simulink model "Starssensegment"  (R2021a)
settings: Solver=VariableStepAuto  StartTime=0.0  StopTime=10  RelTol=1e-3
libraries: simulink x1
settings Model: SnapshotBufferSize=50  SnapshotInterval=50  Creator=timyb  LastModifiedBy=timyb

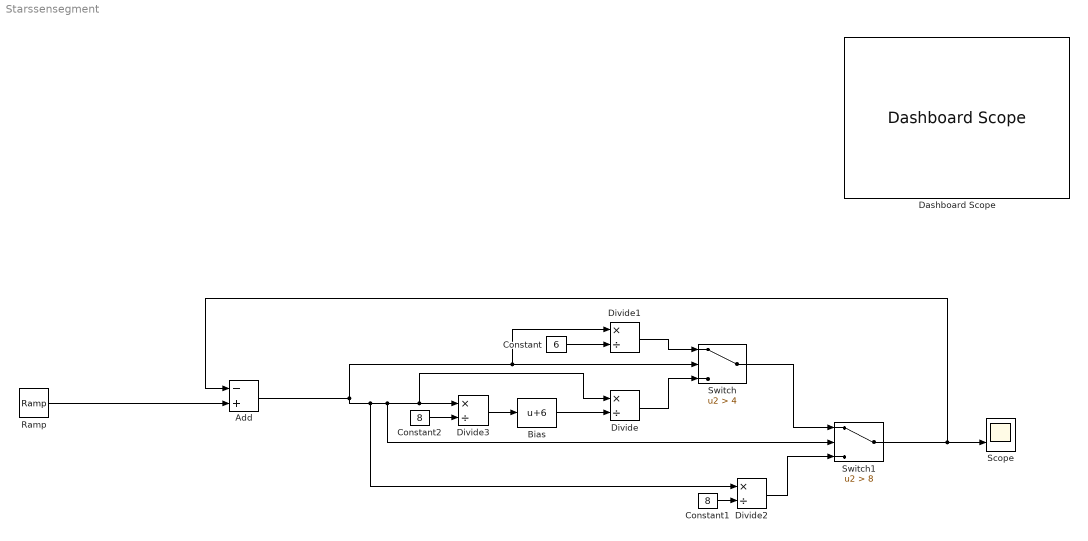
== system Starssensegment ==
  Add : Sum  Inputs=-+
  Bias : Bias  Bias=6
  Constant : Constant  Value=6
  Constant1 : Constant  Value=8
  Constant2 : Constant  Value=8
  Dashboard Scope : DashboardScope
  Divide{,1..3} (4 alike) : Product  Inputs=*/
  Ramp : simulink/Sources/Ramp  slope=0.1  start=0  InitialOutput=0
  Scope : Scope  NumInputPorts=2
  Switch : Switch  Criteria=u2 > Threshold  Threshold=4
  Switch1 : Switch  Criteria=u2 > Threshold  Threshold=8
  wires:
  Add/1 -> Divide2/1, Switch1/2, Divide/1, Divide3/1, Switch/2, Divide1/1
  Bias/1 -> Divide/2
  Divide/1 -> Switch/3
  Constant/1 -> Divide1/2
  Divide1/1 -> Switch/1
  Switch/1 -> Switch1/1
  Constant1/1 -> Divide2/2
  Divide2/1 -> Switch1/3
  Switch1/1 -> Add/1, Scope/2
  Divide3/1 -> Bias/1
  Constant2/1 -> Divide3/2
  Ramp/1 -> Add/2
